simulink model "EcoCAR3_Capstone_P2_LEA_GKN_Enerdel_TheREALone"  (R2014a)
settings: Solver=ode45  StartTime=0.0  StopTime=10.0  RelTol=1e-3
undefined symbols (not defined in the file): chas, DriverControls, EcoCAR3_Lib, eng, eng_plant_init, engine, engine_ratio, ENV, env, fd, gb, gb_ctrl_init, gb_ctrl_trs_init, max_cap, max_cell_curr, motor_ratio, motor_sync_k, motor_sync_Kd, motor_sync_Ki, motor_sync_Kp, num_cell_par, num_cell_series, VEH, veh, veh_plant_init, vpa, vpc, vpc_brake_init, whl, whl_plant_init
libraries: simulink x20, dspsigattribs x1
(part 3 of 3)

== system EcoCAR3_Capstone_P2_LEA_GKN_Enerdel_TheREALone/Architecture/Motor/Controller/Motor Controller/Motor Controller Transient ==
  note: motor_mode
      | 1 = vpc dmd
      | 2 = speed matching
      | 3 = max torque
      | 4 = engine on when driving
      | 5 = motor off
  Motor Mode : Inport
  Powertrain Controller Torque DMD : Inport  Port=2
  GB Gear DMD : Inport  Port=3
  GB SPD Out : Inport  Port=4
  Coupler Torque : Inport  Port=5
  Max Positive Motor Torque : Inport  Port=6
  Max Negative Motor Torque : Inport  Port=7
  ESS Max Power : Inport  Port=8
  Motor SPD : Inport  Port=9
  2-D Lookup Table : Lookup_n-D  BreakpointsForDimension1=[1:3]  BreakpointsForDimension2=[1:3]  InternalRulePriority=Speed  RndMeth=Simplest  InputSameDT=on
  Constant : Constant
  Constant1 : Constant  Value=0
  MinMax : MinMax  Inputs=2
  Multiport Switch : MultiPortSwitch  Inputs=5
  Saturation Dynamic : simulink/Discontinuities/Saturation Dynamic  OutMin=[]  OutMax=[]  OutDataTypeStr=Inherit: Same as second input  OutDataType=fixdt(1, 16)  OutScaling=2^-10  DoSatur=off
  Subsystem : Subsystem
  Switch : Switch  Threshold=0.5
  add : Sum  Inputs=+-
  Motor Controller Transient Value : Outport
  wires:
  Coupler Torque/1 -> add/2
  Powertrain Controller Torque DMD/1 -> Multiport Switch/2, add/1
  Motor SPD/1 -> Subsystem/3(Motor SPD), 2-D Lookup Table/1
  ESS Max Power/1 -> 2-D Lookup Table/2
  Max Positive Motor Torque/1 -> MinMax/1
  2-D Lookup Table/1 -> MinMax/2
  MinMax/1 -> Multiport Switch/4, Saturation Dynamic/1
  Max Negative Motor Torque/1 -> Saturation Dynamic/3
  Multiport Switch/1 -> Motor Controller Transient Value/1
  Saturation Dynamic/1 -> Multiport Switch/3
  Motor Mode/1 -> Subsystem/4(Motor Mode), Switch/2, Switch/1
  Constant/1 -> Switch/3
  Switch/1 -> Multiport Switch/1
  GB Gear DMD/1 -> Subsystem/1(Gear DMD)
  GB SPD Out/1 -> Subsystem/2(Gear SPD Out)
  Subsystem/1(Motor Torque DMD) -> Saturation Dynamic/2
  Constant1/1 -> Multiport Switch/6
  add/1 -> Multiport Switch/5

== system EcoCAR3_Capstone_P2_LEA_GKN_Enerdel_TheREALone/Architecture/Motor/Plant/Motor/Subsystem ==
  motor speed : Inport
  command : Inport  Port=2
  torque : Inport  Port=3
  Abs : Abs
  Add : Sum  Inputs=-+
  Add1 : Sum
  Constant : Constant
  Continuous Prop : Lookup_n-D  NumberOfTableDimensions=1  BreakpointsForDimension1=[-5:5]  Table=tanh([-5:5])  InternalRulePriority=Speed  RndMeth=Simplest  InputSameDT=on
  Continuous Regen : Lookup_n-D  NumberOfTableDimensions=1  BreakpointsForDimension1=[-5:5]  Table=tanh([-5:5])  InternalRulePriority=Speed  RndMeth=Simplest  InputSameDT=on
  Peak Prop : Lookup_n-D  NumberOfTableDimensions=1  BreakpointsForDimension1=[-5:5]  Table=tanh([-5:5])  InternalRulePriority=Speed  RndMeth=Simplest  InputSameDT=on
  Peak Regen : Lookup_n-D  NumberOfTableDimensions=1  BreakpointsForDimension1=[-5:5]  Table=tanh([-5:5])  InternalRulePriority=Speed  RndMeth=Simplest  InputSameDT=on
  Product : Product
  Product1 : Product
  Product2 : Product
  Sign : Signum
  Subsystem : Subsystem
  Switch : Switch
  Switch1 : Switch
  max torque : Outport
  wires:
  Continuous Prop/1 -> Switch/1
  Continuous Regen/1 -> Switch/3
  Peak Prop/1 -> Switch1/1
  Peak Regen/1 -> Switch1/3
  motor speed/1 -> Continuous Prop/1, Continuous Regen/1, Peak Regen/1, Peak Prop/1
  command/1 -> Switch1/2, Switch/2
  Switch/1 -> Product/1, Subsystem/1("continuous torque ")
  torque/1 -> Subsystem/2(torque)
  Subsystem/1(Heat Index) -> Add/1, Product/2
  Constant/1 -> Add/2
  Add/1 -> Product1/1
  Switch1/1 -> Product1/2
  Product/1 -> Add1/1
  Product1/1 -> Add1/2
  Add1/1 -> Sign/1
  Sign/1 -> Abs/1, Product2/1
  Product2/1 -> max torque/1
  Abs/1 -> Product2/2

== system EcoCAR3_Capstone_P2_LEA_GKN_Enerdel_TheREALone/Supervisory Controller/vpc_prop_par_direct_pwr_1mot_pretx/control strategy/Numerics/Electric machine max torque calculation ==
  acc pwr : Inport
  mot trq max regen : Inport  Port=2
  mot trq max prop : Inport  Port=3
  ess pwr max prop : Inport  Port=4
  mc spd : Inport  Port=5
  ess pwr max regen : Inport  Port=6
  MinMax : MinMax  Inputs=2
  MinMax1 : MinMax  Inputs=2
  Motor Inverse torque : Lookup_n-D  BreakpointsForDimension1=mot.plant.calc.trq_pwr_elec.idx1_spd  BreakpointsForDimension2=mot.plant.calc.trq_pwr_elec.idx2_pwr  Table=mot.plant.calc.trq_pwr_elec.map  InternalRulePriority=Speed  RndMeth=Simplest  InputSameDT=on
  Motor Inversetorque : Lookup_n-D  BreakpointsForDimension1=mot.plant.calc.trq_pwr_elec.idx1_spd  BreakpointsForDimension2=mot.plant.calc.trq_pwr_elec.idx2_pwr  Table=mot.plant.calc.trq_pwr_elec.map  InternalRulePriority=Speed  RndMeth=Simplest  InputSameDT=on
  Sum : Sum  Inputs=+-
  Sum1 : Sum  Inputs=+-
  mot_max_elec_trq_pos : Outport
  mot_max_elec_trq_regen : Outport  Port=2
  wires:
  mc spd/1 -> Motor Inversetorque/1, Motor Inverse torque/1
  Motor Inversetorque/1 -> MinMax/1
  mot trq max prop/1 -> MinMax/2
  mot trq max regen/1 -> MinMax1/1
  MinMax1/1 -> mot_max_elec_trq_regen/1
  MinMax/1 -> mot_max_elec_trq_pos/1
  Sum1/1 -> Motor Inverse torque/2
  ess pwr max regen/1 -> Sum1/1
  Sum/1 -> Motor Inversetorque/2
  ess pwr max prop/1 -> Sum/1
  acc pwr/1 -> Sum1/2, Sum/2

== system EcoCAR3_Capstone_P2_LEA_GKN_Enerdel_TheREALone/Supervisory Controller/vpc_prop_par_direct_pwr_1mot_pretx/control strategy/Numerics/Engine torque calculation ==
  whl trq dmd : Inport
  eng trq max : Inport  Port=2
  whl spd : Inport  Port=3
  eng spd : Inport  Port=4
  Soc : Inport  Port=5
  acc pwr : Inport  Port=6
  MinMax : MinMax  Inputs=2
  Product : Product
  Sum : Sum  Inputs=+-+
  ess pwr for SOC regulation : Lookup_n-D  NumberOfTableDimensions=1  BreakpointsForDimension1=vpc.prop.init.ess_pwr_dmd.idx1_soc  Table=vpc.prop.init.ess_pwr_dmd.map  InternalRulePriority=Speed  RndMeth=Simplest  InputSameDT=on
  min = 0 max = inf : Saturate  UpperLimit=inf  LowerLimit=0
  min = eng.plant.init.spd_idle max = inf : Saturate  UpperLimit=inf  LowerLimit=eng.plant.init.spd_idle
  eng_pwr_dmd : Outport
  eng trq dmd : Outport  Port=2
  wires:
  whl trq dmd/1 -> Product/1
  whl spd/1 -> Product/2
  Product/1 -> Sum/1
  ess pwr for SOC regulation/1 -> Sum/2
  acc pwr/1 -> Sum/3
  eng spd/1 -> min = eng.plant.init.spd_idle max = inf/1
  Sum/1 -> eng_pwr_dmd/1
  MinMax/1 -> eng trq dmd/1
  eng trq max/1 -> MinMax/2
  min = 0 max = inf/1 -> MinMax/1

== system EcoCAR3_Capstone_P2_LEA_GKN_Enerdel_TheREALone/Supervisory Controller/vpc_prop_par_direct_pwr_1mot_pretx/control strategy/Numerics/Max torque allowed to avoid sli ==
  vehicle speed : Inport
  gear ratio : Inport  Port=2
  1/whl.plant.init.radius : Gain  Gain=1/whl.plant.init.radius
  Constant : Constant  Value=veh.plant.init.mass*env.init.gravity*chas.plant.init.ratio_weight_front
  Product : Product
  tire friction : Lookup_n-D  NumberOfTableDimensions=1  BreakpointsForDimension1=[-5:5]  Table=tanh([-5:5])  InternalRulePriority=Speed  RndMeth=Simplest  InputSameDT=on
  vpa.calc.eng.ratio_cum : Gain  Gain=vpa.calc.eng.ratio_cum
  Tmax for no slip : Outport
  wires:
  vehicle speed/1 -> tire friction/1
  tire friction/1 -> Product/1
  Constant/1 -> Product/2
  gear ratio/1 -> vpa.calc.eng.ratio_cum/1
  vpa.calc.eng.ratio_cum/1 -> 1/whl.plant.init.radius/1

== system EcoCAR3_Capstone_P2_LEA_GKN_Enerdel_TheREALone/Architecture/Motor/Controller/Motor Controller/Motor Controller Command Map/Subsystem ==
  In1 : Inport
  In2 : Inport  Port=2
  Fcn : Fcn  Expr=u[1]/(u[2]+eps)*(u[2]!=0)
  Mux : Mux  Inputs=2
  Out1 : Outport
  wires:
  In2/1 -> Mux/2
  In1/1 -> Mux/1
  Mux/1 -> Fcn/1
  Fcn/1 -> Out1/1

== system EcoCAR3_Capstone_P2_LEA_GKN_Enerdel_TheREALone/Architecture/Motor/Controller/Motor Controller/Motor Controller Transient/Subsystem ==
  Gear DMD : Inport
  Gear SPD Out : Inport  Port=2
  Motor SPD : Inport  Port=3
  Motor Mode : Inport  Port=4
  Add : Sum  Inputs=+++
  Compare To Constant : simulink/Logic and Bit Operations/Compare To Constant  relop===  const=2  OutDataTypeStr=boolean
  D : Gain  Gain=motor_sync_Kd
  Derivative : Derivative
  Gear Ratio Lookup Table : Lookup_n-D  NumberOfTableDimensions=1  BreakpointsForDimension1=[-5:5]  Table=tanh([-5:5])  InternalRulePriority=Speed  RndMeth=Simplest  InputSameDT=on
  I : Gain  Gain=motor_sync_Ki
  Integrator : Integrator  ExternalReset=rising
  K : Gain  Gain=motor_sync_k
  P : Gain  Gain=motor_sync_Kp
  Product : Product
  Saturation : Saturate  UpperLimit=50  LowerLimit=-50
  Sum : Sum  Inputs=+-
  motor-engine ratio : Gain  Gain=motor_ratio/engine_ratio
  Motor Torque DMD : Outport
  wires:
  Gear DMD/1 -> Gear Ratio Lookup Table/1
  Gear Ratio Lookup Table/1 -> Product/1
  Gear SPD Out/1 -> Product/2
  Product/1 -> motor-engine ratio/1
  motor-engine ratio/1 -> Sum/1
  Motor SPD/1 -> Sum/2
  Sum/1 -> I/1, D/1, P/1
  Motor Mode/1 -> Compare To Constant/1
  I/1 -> Integrator/1
  Compare To Constant/1 -> Integrator/2
  K/1 -> Motor Torque DMD/1
  Add/1 -> K/1
  Integrator/1 -> Add/2
  D/1 -> Derivative/1
  Derivative/1 -> Saturation/1
  Saturation/1 -> Add/3
  P/1 -> Add/1

== system EcoCAR3_Capstone_P2_LEA_GKN_Enerdel_TheREALone/Architecture/Motor/Plant/Motor/Subsystem/Subsystem ==
  "continuous torque " : Inport
  torque : Inport  Port=2
  0.3/mot.plant.init.t_max_trq : Gain
  Abs : Abs
  Add : Sum  Inputs=+-
  Constant : Constant
  Divide : Product  Inputs=*/
  Integrator : Integrator  InitialCondition=-0.3  LimitOutput=on  UpperSaturationLimit=1  LowerSaturationLimit=-0.3
  Saturation : Saturate  UpperLimit=1  LowerLimit=0
  Heat Index : Outport
  wires:
  Divide/1 -> Abs/1
  Constant/1 -> Add/2
  Abs/1 -> Add/1
  Add/1 -> 0.3/mot.plant.init.t_max_trq/1
  0.3/mot.plant.init.t_max_trq/1 -> Integrator/1
  Integrator/1 -> Saturation/1
  Saturation/1 -> Heat Index/1
  "continuous torque "/1 -> Divide/2
  torque/1 -> Divide/1

== stateflow chart EcoCAR3_Capstone_P2_LEA_GKN_Enerdel_TheREALone/Supervisory Controller/vpc_prop_par_direct_pwr_1mot_pretx/control strategy/Chart ==
  state Eng_ON_OFF_Control
    state Eng_OFF
      during:...
      eng_on_dmd=0;
    state Eng_ON_MinTime
      en:
      TStart = t;
      during:...
      eng_on_dmd=1;
    state Eng_OFF_MinTime
      entry:
      TStart = t;
      during:...
      eng_on_dmd=0;
    state Eng_ON
      during:...
      eng_on_dmd=1;
    note: [SOC > vpc_prop_init_eng_soc_ess_above_turn_off && ...
        | MinTimeForEngOff&&(perfo_mode== 0 )&&...
        | whl_trq_dmd/(gb_ratio*vpa_calc_mot_ratio_cum)<...
        | (mot_trq_pos_max*vpc_prop_init_mot_percent_max_low)&&...
        | (accmech_trq== 0 )]
    (default) -> Eng_OFF
    Eng_OFF -> Eng_ON_MinTime : [(SOC <vpc_prop_init_eng_soc_ess_below_turn_on ||...
        | MinTimeForEngOn||perfo_mode||(accmech_trq>0)||...
        | mot_sat_eng_on_dmd==1)&& vpc_prop_init_ev_only==0]
    Eng_OFF_MinTime -> Eng_OFF : [(t-TStart)>=vpc_prop_init_eng_time_min_stay_off ||...
        | (mot_sat_eng_on_dmd==1)||perfo_mode]
    Eng_ON_MinTime -> Eng_ON : [(t-TStart)>=vpc_prop_init_eng_time_min_stay_on ]
    Eng_ON -> Eng_OFF_MinTime
  state Min_OnOffTime
    state EngCanBeOff
    state Min_PwrDmdOff
      entry:
      TCheck = t;
    state EngCanBeOn
    state Min_PwrDmdOn
      entry:
      TCheck = t;
    (default) -> EngCanBeOff
    Min_PwrDmdOff -> EngCanBeOff [order 1] : [(t-TCheck)>vpc_prop_init_eng_time_min_pwr_dmd_below_thresh &&...
        | eng_pwr_dmd<vpc_prop_init_eng_pwr_whl_below_turn_off]
        | {MinTimeForEngOff=1; MinTimeForEngOn=0;}
    EngCanBeOn -> Min_PwrDmdOff : [eng_pwr_dmd<vpc_prop_init_eng_pwr_whl_below_turn_off]
    Min_PwrDmdOff -> EngCanBeOn [order 2] : [eng_pwr_dmd>vpc_prop_init_eng_pwr_whl_below_turn_off]
    Min_PwrDmdOn -> EngCanBeOff [order 1] : [eng_pwr_dmd<vpc_prop_init_eng_pwr_whl_above_turn_on]
        | {MinTimeForEngOn = 0;}
    EngCanBeOff -> Min_PwrDmdOn : [eng_pwr_dmd>vpc_prop_init_eng_pwr_whl_above_turn_on]
    Min_PwrDmdOn -> EngCanBeOn [order 2] : [(t-TCheck)>vpc_prop_init_eng_time_min_pwr_dmd_above_thresh]
        | {MinTimeForEngOn = 1; MinTimeForEngOff=0;}
  state Timer_Performance
    state Perfo_min_time
      entry:
      TCheck_perfo = t;
      perfo_mode=0;
    state Conso_Mode
      during:...
      perfo_mode=0;
    state PerfoOn
      entry: perfo_mode=1;
    (default) -> Perfo_min_time
    Conso_Mode -> Perfo_min_time : [accel_pedal>vpc_prop_init_perfo_thresh_in...
        | && vpc_prop_init_ev_only==0]
    Perfo_min_time -> Conso_Mode [order 1] : [accel_pedal<vpc_prop_init_perfo_thresh_out]
    (junction 53) -> Conso_Mode
    Perfo_min_time -> PerfoOn [order 2] : [(t-TCheck_perfo)>vpc_prop_init_perfo_time_min]
    PerfoOn -> (junction 53) : [accel_pedal<vpc_prop_init_perfo_thresh_out]
  state Torque_Split
    state Stop
      state Engine_On
        during:
        eng_trq_dmd=ml.min(ml.min(eng_pwr_dmd/...
        ml.max(eng_spd,eng_spd_min),eng_trq_max),...
        -mot_trq_regen_max*vpa_calc_mot_ratio_cum/vpa_calc_eng_ratio_cum);
        mot_trq_dmd=mot_trq_dmd_soc_regul;
        mot_sat_eng_on_dmd=0;
      state Engine_Off
        during:
        eng_trq_dmd=0;
        mot_trq_dmd=0;
        mot_sat_eng_on_dmd=0;
      (default) -> Engine_Off
      Engine_Off -> Engine_On : [eng_on_dmd==1 && whl_trq_dmd>-50]
      Engine_On -> Engine_Off : [[eng_on_dmd==0 || whl_trq_dmd>0]]
    state Brake
      entry: eng_trq_dmd=0;
      mot_trq_dmd=0;
    state gb_not_neutral
      state EV
        during:...
        eng_trq_dmd=0;
        prop_state=1;
        state Mc_Norm
          during:...
          mot_trq_dmd=(whl_trq_dmd/(gb_ratio*vpa_calc_mot_ratio_cum));
          mot_sat_eng_on_dmd=0;
        state mot_sat_max_trq_pos
          during:...
          mot_trq_dmd=mot_trq_pos_max;
          mot_sat_eng_on_dmd=1;
        Torque_Split.gb_not_neutral.EV.Mc_Norm -> Torque_Split.gb_not_neutral.EV.mot_sat_max_trq_pos : [whl_trq_dmd/(gb_ratio*vpa_calc_mot_ratio_cum) >...
            |  (mot_trq_pos_max*vpc_prop_init_mot_percent_max)]
        Torque_Split.gb_not_neutral.EV.mot_sat_max_trq_pos -> Torque_Split.gb_not_neutral.EV.Mc_Norm : [whl_trq_dmd/(gb_ratio*vpa_calc_mot_ratio_cum)<...
            | (mot_trq_pos_max*vpc_prop_init_mot_percent_max_low)]
      state HEV
        state Normal_Driving
          state mot_sat_max_trq_regen
            during:...
            mot_trq_dmd=mot_trq_regen_max;
            eng_trq_dmd=ml.min( ...
            (((whl_trq_dmd/(gb_ratio*vpa_calc_mot_ratio_cum) ) +accmech_trq-mot_trq_dmd)*vpa_calc_mot_ratio_cum/vpa_calc_eng_ratio_cum) ...
            , eng_trq_max);
          state Mc_Norm
            during:...
            mot_trq_dmd=mot_trq_eng_opt_dmd;
            eng_trq_dmd=ml.min( ...
            (((whl_trq_dmd/(gb_ratio*vpa_calc_mot_ratio_cum) )+accmech_trq -mot_trq_dmd)*vpa_calc_mot_ratio_cum/vpa_calc_eng_ratio_cum) ...
            , eng_trq_max);
          state mot_sat_max_trq_pos
            during:...
            mot_trq_dmd=mot_trq_pos_max;
            eng_trq_dmd=ml.min( ...
            (((whl_trq_dmd/(gb_ratio*vpa_calc_mot_ratio_cum) ) +accmech_trq-mot_trq_dmd)*vpa_calc_mot_ratio_cum/vpa_calc_eng_ratio_cum) ...
            , eng_trq_max);
          mot_sat_max_trq_regen -> Torque_Split.gb_not_neutral.HEV.Normal_Driving.Mc_Norm : [mot_trq_eng_opt_dmd>(mot_trq_regen_max*vpc_prop_init_mot_percent_max_low)]
          Torque_Split.gb_not_neutral.HEV.Normal_Driving.Mc_Norm -> mot_sat_max_trq_regen [order 1] : [mot_trq_eng_opt_dmd<(mot_trq_regen_max*vpc_prop_init_mot_percent_max)]
          (default) -> Torque_Split.gb_not_neutral.HEV.Normal_Driving.Mc_Norm
          Torque_Split.gb_not_neutral.HEV.Normal_Driving.Mc_Norm -> Torque_Split.gb_not_neutral.HEV.Normal_Driving.mot_sat_max_trq_pos [order 2] : [mot_trq_eng_opt_dmd>(mot_trq_pos_max*vpc_prop_init_mot_percent_max)]
          Torque_Split.gb_not_neutral.HEV.Normal_Driving.mot_sat_max_trq_pos -> Torque_Split.gb_not_neutral.HEV.Normal_Driving.Mc_Norm : [mot_trq_eng_opt_dmd<(mot_trq_pos_max*vpc_prop_init_mot_percent_max_low)]
        state Performance
          during:...
          state Very_Low_SOC
            during:...
            eng_trq_dmd=ml.min(eng_trq_max,trq_max_slip);
            mot_trq_dmd=0;
          state Normal_SOC
            during:...
            eng_trq_dmd=ml.min(eng_trq_max,trq_max_slip);
            mot_trq_dmd=ml.min(mot_trq_pos_max,...
            (trq_max_slip-eng_trq_dmd)/(vpa_calc_mot_ratio_cum/vpa_calc_eng_ratio_cum))
          Normal_SOC -> Very_Low_SOC : [SOC<=ess_plant_init_soc_min]
          Very_Low_SOC -> Normal_SOC : [SOC>ess_plant_init_soc_min]
          (default) -> Normal_SOC
        (default) -> Normal_Driving
        Normal_Driving -> Performance : [perfo_mode]
        Performance -> Normal_Driving : [perfo_mode==0]
      (default) -> EV
      EV -> HEV : [eng_on_dmd==1  && ...
          |  eng_spd>eng_spd_min]
      HEV -> EV : [eng_on_dmd==0]
    state gb_neutral
      during:...
      mot_trq_dmd=0;
      eng_trq_dmd=0;
      prop_state=-1;
      mot_sat_eng_on_dmd=0;
    (default) -> Stop
    Stop -> gb_not_neutral : [whl_trq_dmd>0]
    Brake -> Stop [order 1] : [chas_spd<1]
    Brake -> gb_not_neutral [order 2] : [whl_trq_dmd>0]
    gb_not_neutral -> Brake [order 2] : [whl_trq_dmd <= 0]
    gb_not_neutral -> gb_neutral [order 1] : [gb_ratio==0]
    gb_neutral -> gb_not_neutral : [gb_ratio>0]

== stateflow chart EcoCAR3_Capstone_P2_LEA_GKN_Enerdel_TheREALone/Supervisory Controller/SupervisoryControl/SupervisorLogic ==
  state Drivelogic [parallel]
    settings: executionOrder=1
    state VehicleOfforAcc
    state Shutdown
    state Startup
    state VehicleReady
      state PerformanceDrive
      state NormalDrive
        state EVOnly
          state Accel
          state Brake_Idle
          Drivelogic.VehicleReady.NormalDrive.EVOnly.Accel -> Drivelogic.VehicleReady.NormalDrive.EVOnly.Brake_Idle
          Drivelogic.VehicleReady.NormalDrive.EVOnly.Brake_Idle -> Drivelogic.VehicleReady.NormalDrive.EVOnly.Accel
        state ICEOnly
          state Accel
          state Brake_Idle
        state HEV
          state CD
          state CS
          state Brake_Idle
        EVOnly -> ICEOnly [order 2]
        ICEOnly -> EVOnly [order 2]
        EVOnly -> HEV [order 1]
        HEV -> EVOnly [order 1]
        ICEOnly -> HEV [order 1]
        HEV -> ICEOnly [order 2]
      NormalDrive -> PerformanceDrive
      PerformanceDrive -> NormalDrive
    VehicleOfforAcc -> Startup
    Startup -> VehicleOfforAcc [order 2]
    Shutdown -> VehicleOfforAcc
    VehicleReady -> Shutdown
    Startup -> VehicleReady [order 1]
  state EngineTime [parallel]
    settings: executionOrder=2
  state EngineON [parallel]
    settings: executionOrder=3
  state Clutch [parallel]
    settings: executionOrder=4

== stateflow chart EcoCAR3_Capstone_P2_LEA_GKN_Enerdel_TheREALone/Architecture/Gearbox/Controller/Demand/Gear Shift Logic ==
  state Hold_neutro
    entry: gb_gear_dmd=0:
  state Veh_moving [group]
    state Timer_up
      entry:...
      T_up=t:
    state Up_Shifting
      entry:...
      gb_gear_dmd=gb_gear_last_holded+1;
    state Hold_shift
      entry: gb_gear_last_holded=current_gear:
    state Down_Shifting
      entry:...
      gb_gear_dmd=gb_gear_last_hold-1;
    state Timer_dn
      entry:...
      T_dn=t;
    Timer_up -> (junction 34) [order 2] : [(t-T_up)>gb_ctrl_dmd_init_min_time_for_shift_dmd||acc_cmd==1||...
        | acc_cmd<gb_ctrl_dmd_init_acc_below_no_timer]
    (junction 34) -> (junction 35)
    Timer_up -> Hold_shift [order 1] : [gb_gear_next<=current_gear]
    (junction 27) -> Timer_up : [acc_cmd<1&&acc_cmd>=gb_ctrl_dmd_init_acc_below_no_timer]
    (junction 35) -> (junction 27) [order 2] : [[acc_cmd==1||1acc_cmd<gb_ctrl_dmd_init_acc_below_no_timer]
    Hold_shift -> (junction 27) [order 4] : [gb_gear_next_up>current_gear &&...
        | (gb_spd_in_next_up>gb_spd_in_min||current_gear==0)]
    (junction 35) -> Up_Shifting [order 1]
    Hold_shift -> Up_Shifting [order 2] : [gb_spd_in>gb_spd_in_max&&...
        | current_gear<gb_plant_calc_max]
    Down_Shifting -> Hold_shift : [current_gear==gb_gear_dmd&&(eng_on==0||cpl_lock==1)]
    Up_Shifting -> Hold_shift : [current_gear==gb_gear_dmd&&(eng_on==0||cpl_lock)]
    Hold_shift -> Down_Shifting [order 1] : [gb_spd_in<gb_spd_in_min && current_gear>1]
    Hold_shift -> (junction 21) [order 3]
    Timer_dn -> Hold_shift [order 2] : [gb_gear_next_down>=current_gear]
    (junction 25) -> Down_Shifting
    (junction 21) -> (junction 25) [order 2] : [acc_cmd==1||acc_cmd<gb_ctrl_dmd_init_acc_below_no_timer]
    (junction 26) -> (junction 25)
    (junction 21) -> Timer_dn [order 1] : [acc_cmd<1&&acc_cmd>=gb_ctrl_dmd_int_acc_below_no_timer]
    Timer_dn -> (junction 26) [order 1] : [(t-T_dn)>gb_ctrl_dmd_init_min_time_for_shift_dmd||acc_cmd==1||...
        | acc_cmd<gb_ctrl_dmd_init_acc_below_no_timer]
  (default) -> Hold_neutro
  Hold_neutro -> Veh_moving : [(drv_spd_dmd>0||acc_cmd>0.005)&&...
      | current_gear==gb_gear_dmd]
  Veh_moving -> Hold_neutro : [drv_spd_dmd_decrease == 1 && acc_cmd < 0.005&& chas_spd<gb_ctrl_dmd_init_chas_spd_max_neutro]

== stateflow chart EcoCAR3_Capstone_P2_LEA_GKN_Enerdel_TheREALone/Architecture/Gearbox/Controller/Transient/Gearbox Transient  ==
  note: cpl_mode
      | 1 = cpl open
      | 2 = cpl locked
      | 3 = declutching_fast
      | 4 = reclutching_for_starting
      | 5 = reclutching_slow_for_shifting
      | 6 = reclutching_fast
      |
      | eng_mode
      | 1 = vpc dmd
      | 2 = starting
      | 3 = shifting sync
      | 4 = idling
      | 5= engine off
      |
      | motor_mode
      | 1 = vpc dmd
      | 2 = speed matching
      | 3 = max torque
      | 4 = engine on sync when driving
      | 5 = motor off
  state Stand_by
    note: cpl_mode
        | 1 = cpl open
        | 2 = cpl locked
        | 3 = declutching_fast
        | 4 = reclutching_for_starting
        | 5 = reclutching_slow_for_shifting
        | 6 = reclutching_fast
        |
        | eng_mode
        | 1 = vpc dmd
        | 2 = starting
        | 3 = shifting sync
        | 4 = idling
        | 5= engine off
        |
        | motor_mode
        | 1 = vpc dmd
        | 2 = speed matching
        | 3 = max torque
        | 4 = engine on sync when driving
        | 5 = motor off
    state default
      en: ready_to_go=0;
      veh_mode=1;
    state EV
      en: cpl_mode=1;
      eng_mode=5;
      motor_mode=5;
      ready_to_go=1;
    state HEV
      en: cpl_mode=1;
    state HEV_ready_to_go
      entry: eng_mode=1;
      motor_mode=1;
      ready_to_go=1;
    (default) -> Stand_by.default
    Stand_by.default -> Stand_by.HEV [order 2] : [eng_on == 1]
    Stand_by.default -> Stand_by.EV [order 1] : [eng_on == 0]
    Stand_by.EV -> Stand_by.HEV : [eng_on == 1 && eng_spd>eng_spd_idle]
    Stand_by.HEV -> HEV_ready_to_go : [cpl_position == 0]
    HEV_ready_to_go -> Stand_by.EV : [eng_on == 0]
  state Starting
    note: cpl_mode
        | 1 = cpl open
        | 2 = cpl locked
        | 3 = declutching_fast
        | 4 = reclutching_for_starting
        | 5 = reclutching_slow_for_shifting
        | 6 = reclutching_fast
        |
        | eng_mode
        | 1 = vpc dmd
        | 2 = starting
        | 3 = shifting sync
        | 4 = idling
        | 5= engine off
        |
        | motor_mode
        | 1 = vpc dmd
        | 2 = speed matching
        | 3 = max torque
        | 4 = engine on sync when driving
        | 5 = motor off
    state EV_or_HEV
      en: veh_mode=2;
      trs_finished=0;
      actual_gear==gear_dmd;
    state HEV_locked
      en: cpl_mode=3;
    state EV
      en: cpl_mode = 1;
      motor_mode=1;
    state HEV_unlocked
      en: motor_mode=5;
      eng_mode=2;
      cpl_mode=4;
    state EV_finished
      entry: trs_finished=1;
    state finished
      en: cpl_mode=2;
      eng_mode=1;
      motor_mode=1;
      trs_finished=1;
    (default) -> Starting.EV_or_HEV
    Starting.EV_or_HEV -> Starting.EV [order 1] : [eng_on == 0]
    Starting.EV_or_HEV -> (junction 29) [order 2] : [eng_on ==1]
    (junction 29) -> HEV_locked [order 1] : [cpl_position ==1]
    Starting.EV -> (junction 29) [order 2] : [eng_on == 1]
    (junction 29) -> HEV_unlocked [order 2] : [cpl_position == 0]
    HEV_locked -> HEV_unlocked : [cpl_position == 0]
    Starting.EV -> EV_finished [order 1]
    HEV_unlocked -> finished : [abs(cpl_spd_in - cpl_spd_out)...
        | <cpl_lockup_threshold &&...
        | eng_spd>eng_spd_idle]
  note: 
  state Neutral
    ex: gear_cmd=gear_dmd
    note: cpl_mode
        | 1 = cpl open
        | 2 = cpl locked
        | 3 = declutching_fast
        | 4 = reclutching_for_starting
        | 5 = reclutching_slow_for_shifting
        | 6 = reclutching_fast
        |
        | eng_mode
        | 1 = vpc dmd
        | 2 = starting
        | 3 = shifting sync
        | 4 = idling
        | 5= engine off
        |
        | motor_mode
        | 1 = vpc dmd
        | 2 = speed matching
        | 3 = max torque
        | 4 = engine on sync when driving
        | 5 = motor off
    state default
      en: ready_to_go=0;
      veh_mode=6;
      gear_cmd=0;
    state HEV
      en: cpl_mode=3;
      eng_mode=5;
      motor_mode=5;
    state EV
      en: cpl_mode-1;
      motor_mode=5;
    state HEV_trs_finished
      en: cpl_mode=1;
      eng_mode=4;
      motor_mode=5;
      ready_to_go=1;
    state EV_trs_finished
      en: cpl_mode=1;
      motor_mode=5;
      ready_to_go=1;
    (default) -> Neutral.default
    Neutral.default -> (junction 46) [order 1] : [eng_on_dmd == 0]
    Neutral.default -> (junction 47) [order 2] : [eng_on_dmd == 1]
    (junction 47) -> Neutral.HEV [order 1] : [cpl_position == 1]
    (junction 46) -> Neutral.EV [order 1] : [cpl_position == 1]
    (junction 47) -> HEV_trs_finished [order 2] : [cpl_position == 0]
    (junction 46) -> EV_trs_finished [order 2] : [cpl_position == 0]
    Neutral.HEV -> HEV_trs_finished : [cpl_position == 0]
    Neutral.EV -> EV_trs_finished : [cpl_position == 0]
    HEV_trs_finished -> EV_trs_finished : [eng_on_dmd == 0]
        | {eng_mode=5;}
    EV_trs_finished -> HEV_trs_finished : [eng_on == 1 && eng_spd>eng_spd_idle]
  state Stopping
    note: cpl_mode
        | 1 = cpl open
        | 2 = cpl locked
        | 3 = declutching_fast
        | 4 = reclutching_for_starting
        | 5 = reclutching_slow_for_shifting
        | 6 = reclutching_fast
        |
        | eng_mode
        | 1 = vpc dmd
        | 2 = starting
        | 3 = shifting sync
        | 4 = idling
        | 5= engine off
        |
        | motor_mode
        | 1 = vpc dmd
        | 2 = speed matching
        | 3 = max torque
        | 4 = engine on sync when driving
        | 5 = motor off
    state EV_or_HEV
      en: veh_mode=5;
      trs_finished=0;
    state EV
      en: cpl_mode=1;
    state HEV
      en: cpl_mode=1;
      eng_mode=4;
    (default) -> Stopping.EV_or_HEV
    Stopping.EV_or_HEV -> Stopping.EV [order 1] : [eng_on == 0]
    Stopping.EV_or_HEV -> Stopping.HEV [order 2] : [eng_on == 1]
  state Drving
    note: cpl_mode
        | 1 = cpl open
        | 2 = cpl locked
        | 3 = declutching_fast
        | 4 = reclutching_for_starting
        | 5 = reclutching_slow_for_shifting
        | 6 = reclutching_fast
        |
        | eng_mode
        | 1 = vpc dmd
        | 2 = starting
        | 3 = shifting sync
        | 4 = idling
        | 5= engine off
        |
        | motor_mode
        | 1 = vpc dmd
        | 2 = speed matching
        | 3 = max torque
        | 4 = engine on sync when driving
        | 5 = motor off
    state EV_or_HEV
      en: veh_mode=3;
    state HEV
      en: cpl_mode=2;
      eng_mode=1;
      shifting_ready=1;
      motor_mode=1;
    state EV
      en: cpl_mode=1;
      shifting_ready=1;
      motor_mode=1;
    state clutching
      en: cpl_mode=5;
      motor_mode=4;
    state eng_sync
      en: eng_mode=3;
      shifting_ready=0;
    (default) -> Drving.EV_or_HEV
    Drving.EV_or_HEV -> Drving.EV [order 1] : [eng_on == 0]
    Drving.EV_or_HEV -> Drving.HEV [order 2] : [eng_on == 1]
    Drving.HEV -> Drving.EV : [eng_on == 0]
    Drving.EV -> eng_sync : [eng_on == 1]
    clutching -> Drving.HEV : [abs(cpl_spd_in - cpl_spd_out)...
        |  < cpl_lockup_threshold]
    eng_sync -> clutching : [eng_spd > eng_spd_idle && abs(cpl_spd_in - cpl_spd_out) < cpl_clutching_threshold]
  state Shifting
    note: cpl_mode
        | 1 = cpl open
        | 2 = cpl locked
        | 3 = declutching_fast
        | 4 = reclutching_for_starting
        | 5 = reclutching_slow_for_shifting
        | 6 = reclutching_fast
        |
        | eng_mode
        | 1 = vpc dmd
        | 2 = starting
        | 3 = shifting sync
        | 4 = idling
        | 5= engine off
        |
        | motor_mode
        | 1 = vpc dmd
        | 2 = speed matching
        | 3 = max torque
        | 4 = engine on sync when driving
        | 5 = motor off
    state EV_orHEV1
      en: veh_mode=4;
      trs_finished=0;
    state EV1
      en:shift_in_prog=1;
      gear_cmd=gear_dmd;
      motor_mode=2;
      time_trs=t;
    state HEV1
      en: shift_in_prog=1;
      gear_cmd=gear_dmd;
      eng_mode=3;
      motor_mode=2;
      cpl_mode=2;
      time_trs=t;
    state finish_EV
      en:shift_in_prog=0;
      trs_finished=1;
      previous_gear=actual_gear;
      motor_mode=1;
    state finish_HEV
      entry: shift_in_prog=0;
      eng_mode=1;
      motor_mode=1;
      trs_finished=1;
      previous_gear=actual_gear;
    (default) -> EV_orHEV1
    EV_orHEV1 -> EV1 [order 2] : [eng_on == 0]
    EV_orHEV1 -> HEV1 [order 1] : [eng_on ==1]
    HEV1 -> finish_HEV : [t - time_trs > shift_time &&...
        | actual_gear == gear_dmd]
    EV1 -> finish_EV : [t - time_trs > shift_time &&...
        | actual_gear == gear_dmd]
  (junction 107) -> Starting
  (default) -> Stand_by
  (junction 105) -> (junction 107) [order 1] : [accel_dmd > 0]
  Stand_by -> (junction 90) : [ready_to_go == 1 &&...
      | gear_dmd > 0 &&...
      | accel_dmd >  accel_stop_threshold]
  (junction 90) -> Starting
  (junction 129) -> Stand_by
  (junction 91) -> (junction 90) [order 1] : [veh_spd <...
      | veh_spd_begin_stopping]
  Neutral -> (junction 129) [order 2] : [veh_spd <= veh_stop_threshold]
  Starting -> (junction 120) [order 3] : [gear_dmd == 0]
      | {cpl_mode = 1; eng_mode = 4; motot_mode = 5;}
  (junction 120) -> (junction 123)
  Stopping -> Stand_by [order 2] : [veh_spd <= veh_stop_threshold]
  Starting -> Stopping [order 2] : [gear_dmd == 0 ||...
      | accel_dmd == 0]
  Starting -> Drving [order 1] : [trs_finihsed == 1]
  (junction 105) -> Stopping [order 2] : [accel_dmd <= 0]
  (junction 106) -> (junction 105) [order 1] : [veh_spd <...
      | veh_spd_begin_stopping]
  Stopping -> (junction 91) [order 1] : [accel_dmd > accel_stop_threshold &&...
      | gear_dmd > 0]
  (junction 91) -> Drving [order 2] : [veh_spd >=...
      | veh_spd_begin_stiopping]
  Drving -> Shifting [order 1] : [shifting-ready == 1 &&...
      | gear_dmd ~= actual_gear &&...
      | gear_dmd > 0]
  Shifting -> Drving : [trs_finished == 1]
  Drving -> Stopping [order 2] : [veh_spd < veh_spd_begin_stopping &&...
      | accel_dmd <= accel_stop_threshold]
  Neutral -> (junction 106) [order 1] : [ready_to_go ==1 &&...
      | gear_dmd > 0]
  (junction 106) -> Drving [order 2] : [veh_spd > veh_spd_begin_stopping]
  (junction 126) -> Neutral
  Stopping -> (junction 114) [order 3] : [gear_dmd == 0]
  Drving -> (junction 117) [order 3] : [gear_dmd == 0]
  (junction 114) -> (junction 126)
  (junction 117) -> (junction 114)
  (junction 123) -> (junction 117)
  data: eng_on_dmd input; eng_on input; eng_spd input; cpl_spd_in input; cpl_spd_out input; cpl_position input; eng_mode output; motor_mode output; cpl_mode output; shift_in_prog output; veh_mode output; gear_cmd output; previous_gear output; gear_dmd input; actual_gear input; accel_dmd input; veh_spd input; eng_spd_idle input; eng_stop_threshold input; veh_spd_begin_stopping input; veh_spd_started input; cpl_lockup_threshold input; cpl_clutching_threshold input; accel_stop_threshold input; shift_time input

== stateflow chart EcoCAR3_Capstone_P2_LEA_GKN_Enerdel_TheREALone/Architecture/Engine/Plant1/Chart ==
  state Engine_On
    state Fuel_On
      during:...
      eng_trq_out=((1-trq_cmd)*min_eng_trq)+(trq_cmd*max_eng_trq);
    (default) -> Fuel_On
  state Engine_OFF
    during:...
    eng_trq_out=eng_trq_eng_off;
  (default) -> Engine_On
  Engine_On -> Engine_OFF : [eng_on=0|| ...
      | eng_spd<=stall_spd]
  Engine_OFF -> Engine_On : [eng_on=0&& ...
      | eng_spd>1.1*stall_spd]
  data: eng_on input; eng_spd input; trq_cmd input; eng_trq_out output; max_eng_trq input; min_eng_trq input; eng_trq_eng_off input; stall_spd input

== stateflow chart EcoCAR3_Capstone_P2_LEA_GKN_Enerdel_TheREALone/Architecture/Engine/Plant1/Chart1 ==
  state fuel_off
    during:...
    fuel_rate_out=0;
  state fuelling
    during:...
    fuel_rate_out = fuel_rate_in;
  (default) -> fuelling
  fuelling -> fuel_off : [eng_on == 0|| ...
      | eng_spd<stall_spd]
  fuel_off -> fuelling : [eng_on == 1|| ...
      | eng_spd>stall_spd]
  data: fuel_rate_in input; fuel_rate_out output; eng_on input; stalll_spd input; eng_spd input

== stateflow chart EcoCAR3_Capstone_P2_LEA_GKN_Enerdel_TheREALone/Supervisory Controller/Subsystem/SupervisoryLogicChart ==
  state VehReady
    en: powerMode = 2;
    du: hydBrkReq_percent = BPP_percent;
    state EvOnly
      en:engTrqReq_percent = 0;
      state EV_Mode
        du: motTrqReq_percent = APP_percent;
      state Braking
        du:motTrqReq_percent= -min(100,5*BPP_percent*regenFactor);
      (default) -> EV_Mode
      VehReady.EvOnly.Braking -> EV_Mode : [APP_percent > 2 &&...
          | BPP_percent < 2]
      EV_Mode -> VehReady.EvOnly.Braking : [APP_percent < 1 ||...
          | BPP_percent > 1]
    state EngOnly
      en: motTrqReq_percent = 0;
      du:
      engOnReq = 1;
      engTrqReq_percent = APP_percent;
    state EngBlend
      en:
      engOnReq = 1;
      state Propel
        state rtmDrag
          du:
          engTrqReq_percent = APP_percent+motDrag_percent;
          motTrqReq_percent = -motDrag_percent;
        state iceLaunch
          du:
          engTrqReq_percent = 0;
          motTrqReq_percent = APP_percent;
        (default) -> iceLaunch
        iceLaunch -> rtmDrag : [vehVel_mph > 20]
        rtmDrag -> iceLaunch : [vehVel_mph < 15]
      state Braking
        du:
        engTrqReq_percent = 0;
        motTrqReq_percent= -min(100,5*BPP_percent*regenFactor);
      VehReady.EngBlend.Braking -> Propel : [APP_percent > 2 &&...
          | BPP_percent < 2]
      Propel -> VehReady.EngBlend.Braking : [APP_percent < 1 ||...
          | BPP_percent > 1]
      (default) -> VehReady.EngBlend.Braking
    (default) -> EvOnly
    EvOnly -> EngOnly [order 1] : [(essSOC_0_1 < .02 && ...
        | iceSystemStatus == 2) || ...
        | eSystemStatus == 0]
    EngOnly -> EvOnly [order 1] : [(essSOC_0_1 > .24 && ...
        | eSystemStatus == 2) || ...
        | iceSystemStatus == 0]
    EngOnly -> EngBlend [order 2] : [essSOC_0_1 >= .05 && ...
        | iceSystemStatus == 2 && ...
        | eSystemStatus == 2]
    EngBlend -> EngOnly [order 1] : [(essSOC_0_1 < .02 && ...
        | iceSystemStatus == 2) || ...
        | eSystemStatus == 0]
    EvOnly -> EngBlend [order 2] : [essSOC_0_1 <= .20 && ...
        | iceSystemStatus == 2 && ...
        | eSystemStatus == 2]
    EngBlend -> EvOnly [order 2] : [(essSOC_0_1 > .22 && ...
        | eSystemStatus == 2) || ...
        | iceSystemStatus == 0]
  state VehOn
    en: powerMode=1;
    en: closeContactorsReq = 1;
  state VehShutdown
    en: powerMode=2;
    du:motTrqReq_percent=0;
    en: closeContactorsReq = 0;
  state VehOffOrAcc
    en: powerMode=0;
  VehOn -> VehReady [order 2] : [keyPos>=2]
  VehReady -> VehShutdown : [keyPos<2]
  VehShutdown -> VehOffOrAcc : after(1,sec)
  VehOffOrAcc -> VehOn : [keyPos>=1]
  VehOn -> VehOffOrAcc [order 1] : [keyPos<1]
  (default) -> VehOffOrAcc
  data: eSystemStatus input double; iceSystemStatus input; APP_percent input double; BPP_percent input double; keyPos input double; motTrqReq_percent output double; engTrqReq_percent output double; hydBrkReq_percent output double; powerMode output double; closeContactorsReq output double; engOnReq output boolean; ChartMode output Enum: ChartModeType; vehVel_mph input double; regenFactor input double; essSOC_0_1 input; motDrag_percent input
